simulink model "test_org"  (Simulink 10.0)
settings: Solver=ode45  StartTime=0.0  StopTime=1000  MaxStep=1e-3  RelTol=1e-12  AbsTol=1e-12  EnableMultiTasking=on
undefined symbols (not defined in the file): water_level, water_model, WaterRunner_lib
settings Model: Creator=Metti  LastModifiedBy=bhisma
settings SolverCC: AutoScaleAbsTol=off  ZeroCrossControl=DisableAll
settings DataIOCC: LimitDataPoints=on
settings OptimizationCC: ExpressionDepthLimit=2147483647
settings DebuggingCC: SolverPrmCheckMsg=warning  StateNameClashWarn=warning
settings GRTTargetCC: GeneratePreprocessorConditionals=Disable all  CombineOutputUpdateFcns=on  GRTInterface=off
settings ConfigComp: CovExternalEMLEnable=off
settings SimscapeCC: SimscapeNormalizeSystem=off
settings ConfigurationSet: Description=SimMechanics 2G

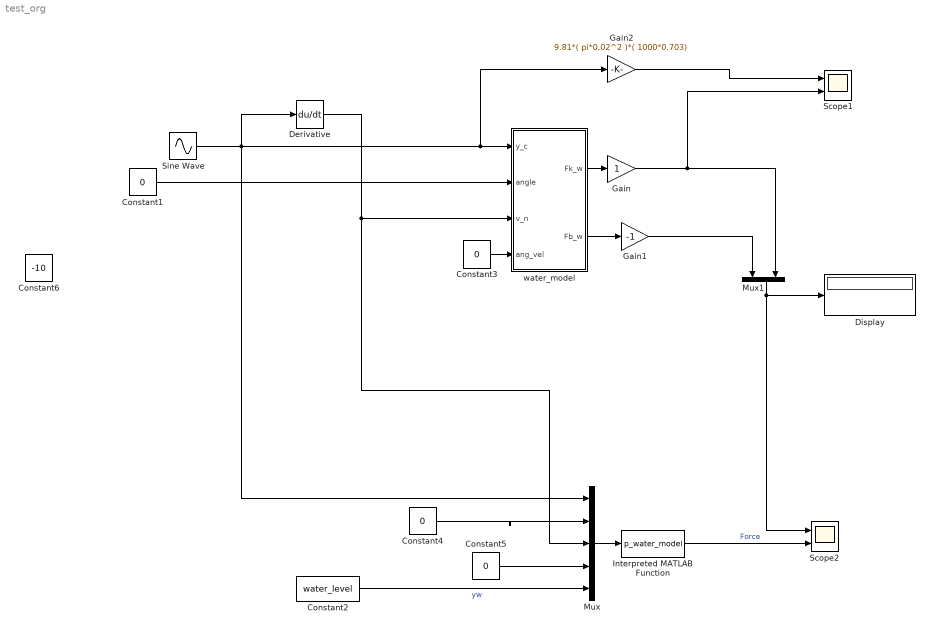
== system test_org ==
  Constant{1,3..5} (4 alike) : Constant  Value=0
  Constant2 : Constant  Value=water_level
  Constant6 : Constant  Value=-10
  Derivative : Derivative
  Display : Display
  Gain : Gain
  Gain1 : Gain  Gain=-1
  Gain2 : Gain  Gain=9.81*( pi*0.02^2 )*( 1000*0.703)
  Interpreted MATLAB Function : MATLABFcn  MATLABFcn=p_water_model  OutputDimensions=2
  Mux : Mux  Inputs=5
  Mux1 : Mux  Inputs=2
  Scope1 : Scope  NumInputPorts=2
  Scope2 : Scope  NumInputPorts=2
  Sine Wave : Sin  Amplitude=0.03  Frequency=50  SampleTime=0
  water_model : Subsystem  AncestorBlock=WaterRunner_lib/water_model  mask{Cd=0.703, density=1000, y_w=water_level, R=0.02, g=-9.81}
      mask prompts: Cd "Drag Coefficient"; y_w "Water level"; R "Foot Radius"; g "Gravity constant (use negative)"
  wires:
  water_model/1(Fk_w) -> Gain/1
  water_model/2(Fb_w) -> Gain1/1
  Mux/1 -> Interpreted MATLAB Function/1
  Interpreted MATLAB Function/1 -> Scope2/2  "Force"
  Mux1/1 -> Display/1, Scope2/1
  Sine Wave/1 -> Derivative/1, Gain2/1, water_model/1(y_c), Mux/1
  Constant1/1 -> water_model/2(angle)
  Constant3/1 -> water_model/4(ang_vel)
  Constant4/1 -> Mux/2
  Gain/1 -> Scope1/2, Mux1/2
  Gain1/1 -> Mux1/1
  Constant5/1 -> Mux/4
  Gain2/1 -> Scope1/1
  Constant2/1 -> Mux/5  "yw"
  Derivative/1 -> Mux/3, water_model/3(v_n)

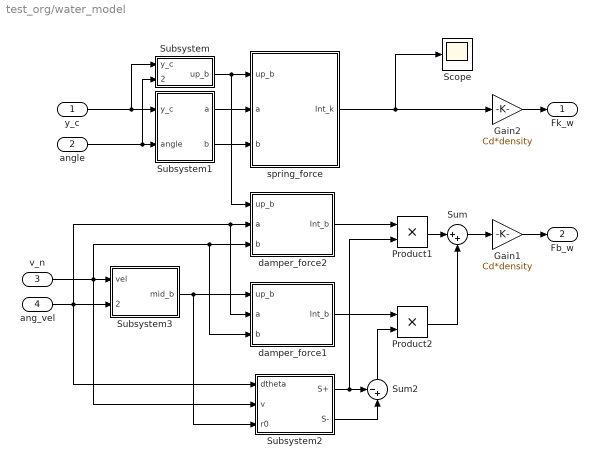
== system test_org/water_model ==
  y_c : Inport
  angle : Inport  Port=2
  v_n : Inport  Port=3
  ang_vel : Inport  Port=4
  Gain1 : Gain  Gain=Cd*density
  Gain2 : Gain  Gain=Cd*density
  Product1 : Product  RndMeth=Zero
  Product2 : Product  RndMeth=Zero
  Scope : Scope
  Subsystem : Subsystem
  Subsystem1 : Subsystem
  Subsystem2 : Subsystem
  Subsystem3 : Subsystem
  Sum : Sum  Inputs=|++
  Sum2 : Sum  Inputs=-+|
  damper_force1 : Subsystem
  damper_force2 : Subsystem
  spring_force : Subsystem
  Fk_w : Outport
  Fb_w : Outport  Port=2
  wires:
  Subsystem3/1(mid_b) -> Subsystem2/3(r0), damper_force1/1(up_b)
  Sum2/1 -> Product2/2
  Subsystem2/2(S-) -> Sum2/2
  Subsystem2/1(S+) -> Product1/2, Sum2/1
  damper_force1/1(Int_b) -> Product2/1
  damper_force2/1(Int_b) -> Product1/1
  Product1/1 -> Sum/1
  Subsystem/1(up_b) -> spring_force/1(up_b), damper_force2/1(up_b)
  y_c/1 -> Subsystem1/1(y_c), Subsystem/1(y_c)
  angle/1 -> Subsystem1/2(angle), Subsystem/2(angle)
  Subsystem1/1(a) -> spring_force/2(a)
  v_n/1 -> Subsystem2/2(v), Subsystem3/1(vel), damper_force2/3(b), damper_force1/3(b)
  ang_vel/1 -> Subsystem2/1(dtheta), Subsystem3/2(dtheta), damper_force2/2(a), damper_force1/2(a)
  Gain2/1 -> Fk_w/1
  spring_force/1(Int_k) -> Gain2/1, Scope/1
  Subsystem1/2(b) -> spring_force/3(b)
  Product2/1 -> Sum/2
  Sum/1 -> Gain1/1
  Gain1/1 -> Fb_w/1

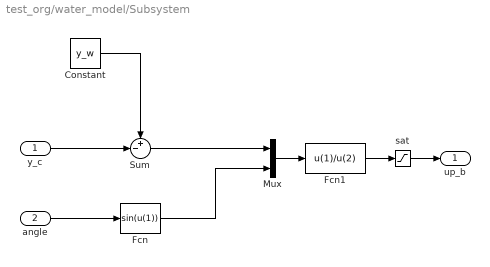
== system test_org/water_model/Subsystem ==
  y_c : Inport
  angle : Inport  Port=2
  Constant : Constant  Value=y_w
  Fcn : Fcn  Expr=sin(u(1))
  Fcn1 : Fcn  Expr=u(1)/u(2)
  Mux : Mux  Inputs=2
  Sum : Sum  Inputs=+-|
  sat : Saturate  UpperLimit=R  LowerLimit=-R
  up_b : Outport
  wires:
  sat/1 -> up_b/1
  Fcn/1 -> Mux/2
  Mux/1 -> Fcn1/1
  Constant/1 -> Sum/1
  y_c/1 -> Sum/2
  Fcn1/1 -> sat/1
  angle/1 -> Fcn/1
  Sum/1 -> Mux/1

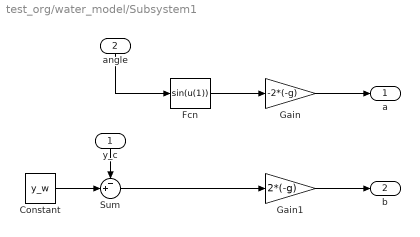
== system test_org/water_model/Subsystem1 ==
  y_c : Inport
  angle : Inport  Port=2
  Constant : Constant  Value=y_w
  Fcn : Fcn  Expr=sin(u(1))
  Gain : Gain  Gain=-2*(-g)
  Gain1 : Gain  Gain=2*(-g)
  Sum : Sum  Inputs=-+|
  a : Outport
  b : Outport  Port=2
  wires:
  Gain1/1 -> b/1
  Gain/1 -> a/1
  Fcn/1 -> Gain/1
  Constant/1 -> Sum/2
  Sum/1 -> Gain1/1
  y_c/1 -> Sum/1
  angle/1 -> Fcn/1

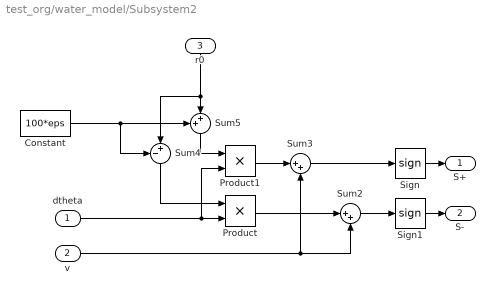
== system test_org/water_model/Subsystem2 ==
  dtheta : Inport
  v : Inport  Port=2
  r0 : Inport  Port=3
  Constant : Constant  Value=100*eps
  Product : Product  RndMeth=Zero
  Product1 : Product  RndMeth=Zero
  Sign : Signum
  Sign1 : Signum
  Sum2 : Sum  Inputs=|++
  Sum3 : Sum  Inputs=|++
  Sum4 : Sum  Inputs=-+|
  Sum5 : Sum  Inputs=++|
  S+ : Outport
  S- : Outport  Port=2
  wires:
  Sum2/1 -> Sign1/1
  Sum3/1 -> Sign/1
  Constant/1 -> Sum5/1, Sum4/1
  Sum4/1 -> Product/1
  v/1 -> Sum3/2, Sum2/2
  Sign/1 -> S+/1
  dtheta/1 -> Product1/2, Product/2
  r0/1 -> Sum5/2, Sum4/2
  Sign1/1 -> S-/1
  Sum5/1 -> Product1/1
  Product1/1 -> Sum3/1
  Product/1 -> Sum2/1

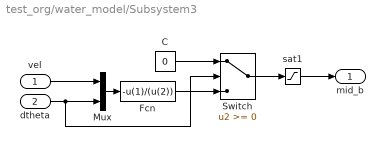
== system test_org/water_model/Subsystem3 ==
  vel : Inport
  dtheta : Inport  Port=2
  C : Constant  Value=0
  Fcn : Fcn  Expr=-u(1)/(u(2))
  Mux : Mux  Inputs=2
  Switch : Switch
  sat1 : Saturate  UpperLimit=R  LowerLimit=-R
  mid_b : Outport
  wires:
  Mux/1 -> Fcn/1
  dtheta/1 -> Switch/2, Mux/2
  vel/1 -> Mux/1
  sat1/1 -> mid_b/1
  Fcn/1 -> Switch/3
  Switch/1 -> sat1/1
  C/1 -> Switch/1

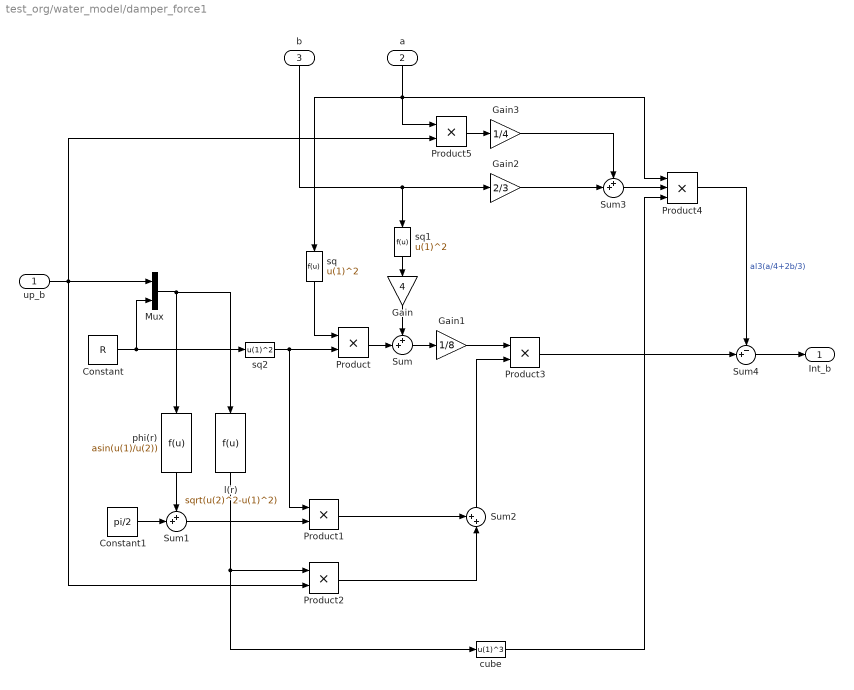
== system test_org/water_model/damper_force1 ==
  up_b : Inport
  a : Inport  Port=2
  b : Inport  Port=3
  Constant : Constant  Value=R
  Constant1 : Constant  Value=pi/2
  Gain : Gain  Gain=4
  Gain1 : Gain  Gain=1/8
  Gain2 : Gain  Gain=2/3
  Gain3 : Gain  Gain=1/4
  Mux : Mux  Inputs=2
  Product{,1..3,5} (5 alike) : Product  RndMeth=Zero
  Product4 : Product  Inputs=3  RndMeth=Zero
  Sum{,1..3} (4 alike) : Sum  Inputs=++|
  Sum4 : Sum  Inputs=-+|
  cube : Fcn  Expr=u(1)^3
  l(r) : Fcn  Expr=sqrt(u(2)^2-u(1)^2)
  phi(r) : Fcn  Expr=asin(u(1)/u(2))
  sq : Fcn  Expr=u(1)^2
  sq1 : Fcn  Expr=u(1)^2
  sq2 : Fcn  Expr=u(1)^2
  Int_b : Outport
  wires:
  Product5/1 -> Gain3/1
  b/1 -> sq1/1, Gain2/1
  a/1 -> sq/1, Product4/1, Product5/1
  Constant/1 -> Mux/2, sq2/1
  sq/1 -> Product/1
  sq1/1 -> Gain/1
  Gain/1 -> Sum/1
  Product/1 -> Sum/2
  Sum/1 -> Gain1/1
  up_b/1 -> Mux/1, Product2/2, Product5/2
  Mux/1 -> l(r)/1, phi(r)/1
  phi(r)/1 -> Sum1/1
  Constant1/1 -> Sum1/2
  Sum1/1 -> Product1/2
  sq2/1 -> Product1/1, Product/2
  l(r)/1 -> cube/1, Product2/1
  Product1/1 -> Sum2/1
  Product2/1 -> Sum2/2
  Gain1/1 -> Product3/1
  Sum2/1 -> Product3/2
  Gain2/1 -> Sum3/2
  Gain3/1 -> Sum3/1
  Sum3/1 -> Product4/2
  cube/1 -> Product4/3
  Product3/1 -> Sum4/2
  Product4/1 -> Sum4/1  "al3(a/4+2b/3)"
  Sum4/1 -> Int_b/1

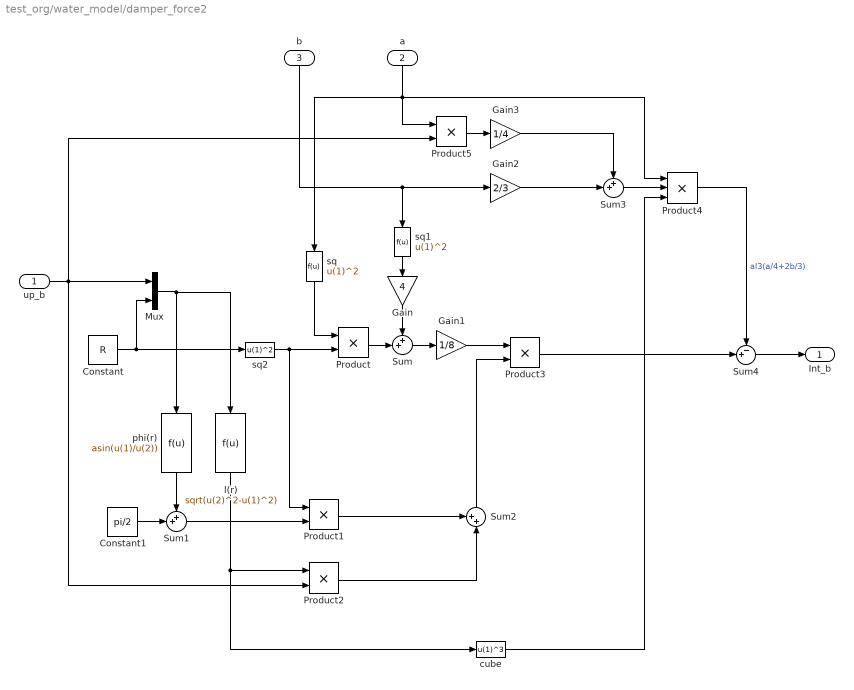
== system test_org/water_model/damper_force2 ==
  up_b : Inport
  a : Inport  Port=2
  b : Inport  Port=3
  Constant : Constant  Value=R
  Constant1 : Constant  Value=pi/2
  Gain : Gain  Gain=4
  Gain1 : Gain  Gain=1/8
  Gain2 : Gain  Gain=2/3
  Gain3 : Gain  Gain=1/4
  Mux : Mux  Inputs=2
  Product{,1..3,5} (5 alike) : Product  RndMeth=Zero
  Product4 : Product  Inputs=3  RndMeth=Zero
  Sum{,1..3} (4 alike) : Sum  Inputs=++|
  Sum4 : Sum  Inputs=-+|
  cube : Fcn  Expr=u(1)^3
  l(r) : Fcn  Expr=sqrt(u(2)^2-u(1)^2)
  phi(r) : Fcn  Expr=asin(u(1)/u(2))
  sq : Fcn  Expr=u(1)^2
  sq1 : Fcn  Expr=u(1)^2
  sq2 : Fcn  Expr=u(1)^2
  Int_b : Outport
  wires:
  Sum4/1 -> Int_b/1
  Product4/1 -> Sum4/1  "al3(a/4+2b/3)"
  Product3/1 -> Sum4/2
  cube/1 -> Product4/3
  Sum3/1 -> Product4/2
  Gain3/1 -> Sum3/1
  Gain2/1 -> Sum3/2
  Sum2/1 -> Product3/2
  Gain1/1 -> Product3/1
  Product2/1 -> Sum2/2
  Product1/1 -> Sum2/1
  l(r)/1 -> Product2/1, cube/1
  sq2/1 -> Product/2, Product1/1
  Sum1/1 -> Product1/2
  Constant1/1 -> Sum1/2
  phi(r)/1 -> Sum1/1
  Mux/1 -> phi(r)/1, l(r)/1
  up_b/1 -> Product5/2, Product2/2, Mux/1
  Sum/1 -> Gain1/1
  Product/1 -> Sum/2
  Gain/1 -> Sum/1
  sq1/1 -> Gain/1
  sq/1 -> Product/1
  Constant/1 -> sq2/1, Mux/2
  a/1 -> Product5/1, Product4/1, sq/1
  b/1 -> Gain2/1, sq1/1
  Product5/1 -> Gain3/1

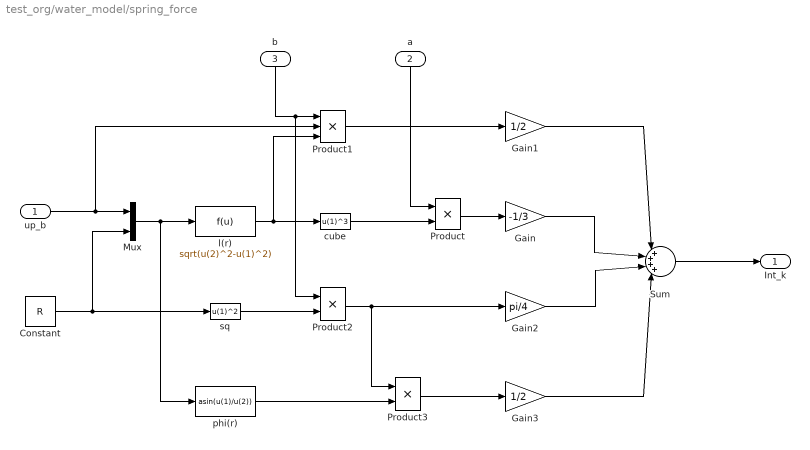
== system test_org/water_model/spring_force ==
  up_b : Inport
  a : Inport  Port=2
  b : Inport  Port=3
  Constant : Constant  Value=R
  Gain : Gain  Gain=-1/3
  Gain1 : Gain  Gain=1/2
  Gain2 : Gain  Gain=pi/4
  Gain3 : Gain  Gain=1/2
  Mux : Mux  Inputs=2
  Product : Product  RndMeth=Zero
  Product1 : Product  Inputs=3  RndMeth=Zero
  Product2 : Product  RndMeth=Zero
  Product3 : Product  RndMeth=Zero
  Sum : Sum  Inputs=|++++|
  cube : Fcn  Expr=u(1)^3
  l(r) : Fcn  Expr=sqrt(u(2)^2-u(1)^2)
  phi(r) : Fcn  Expr=asin(u(1)/u(2))
  sq : Fcn  Expr=u(1)^2
  Int_k : Outport
  wires:
  Product2/1 -> Gain2/1, Product3/1
  sq/1 -> Product2/2
  a/1 -> Product/1
  l(r)/1 -> cube/1, Product1/3
  Product1/1 -> Gain1/1
  Constant/1 -> sq/1, Mux/2
  Mux/1 -> l(r)/1, phi(r)/1
  up_b/1 -> Mux/1, Product1/2
  Product/1 -> Gain/1
  phi(r)/1 -> Product3/2
  Gain1/1 -> Sum/1
  Gain3/1 -> Sum/4
  Sum/1 -> Int_k/1
  Gain/1 -> Sum/2
  Gain2/1 -> Sum/3
  Product3/1 -> Gain3/1
  b/1 -> Product1/1, Product2/1
  cube/1 -> Product/2
